simulink library "lib_ares"  (R2020a)
settings: Solver=VariableStepAuto  StartTime=0.0  StopTime=10.0  RelTol=1e-3
undefined symbols (not defined in the file or in its folder): DiscIntNeverNeededParam
libraries: simulink x9, $bdroot x6
(part 1 of 2)
settings Model: Creator=geiger_br  LastModifiedBy=geiger_br

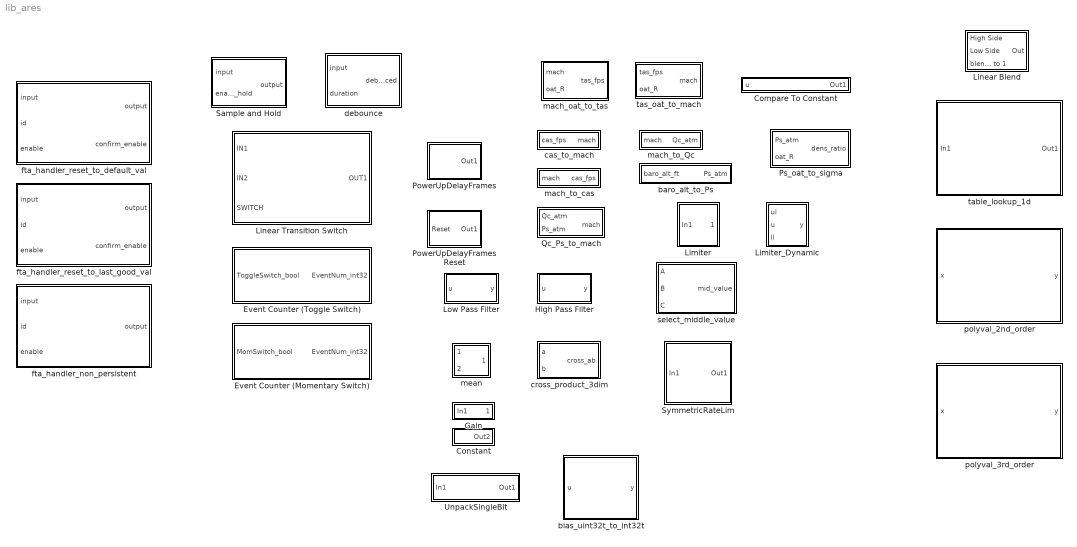
== system lib_ares ==
  Compare To Constant : Subsystem  mask{constval=0}
      mask prompts: constval "Constant:"
      mask init:
      | % Get the mask object
      | mo = get_param(gcb,'MaskObject');
      | % Get the text object
      | % tc = mo.getDialogControl('TextControl');
      | % Change the string
      | % tc.Prompt = mo.Parameters(1).Value;
      | 
      | prm_str = mo.Parameters(1).Value;
      mask Display:
      | if isnan(str2double(prm_str))
      |     fprintf('== %s (%d)',prm_str,int32(constval));
      | else
      |     fprintf('== %g',constval);
      | end
  Constant : Subsystem  mask(Custom Gain Block){const_param=1, const_datatype_str=Inherit: Inherit from 'Constant value', use_attr_fmt_str=on}
      mask prompts: const_param "Gain"; const_datatype_str "Data Type"; use_attr_fmt_str "Use Attributes Format String"
      mask help: Multiply the incoming signal by the gain value.
      mask init:
      | %
      | % NOTES
      | %    For this to work properly, 'Evaluate' must be off for const_param
      | %    The block evaluates here in initialization.
      | %
      | % int64 and uint64 types have been turned off in the Data Type option to
      | % ensure backwards compatibility with R2017a
      | %
      | 
      | evconst = evalin('base',const_param);
      | 
      | % get the mask object data
      | mo = get_param(gcb,'MaskObject');
      | 
      | % Check to see if this is a Parameter.
      | if strcmp(class(evconst),'Simulink.Parameter')
      |     is_parameter = true;
      |     const_value = evconst.Value;
      |     dtype = evconst.DataType;
      |     mo.Parameters(2).Enabled = 'off';
      |     mo.Parameters(2).Value = dtype;
      | else
      |     is_parameter = false;
      |     const_value = evconst;
      | %     dtype='Inherit: Inherit via internal rule';
      |     dtype = mo.Parameters(2).Value;
      |     mo.Parameters(2).Enabled = 'on';
      | end
      | 
      | % Set the gain block to the desired output datatype
      | set_param([gcb '/constant_value'],'OutDataTypeStr',dtype)
      | 
      | % Get the text of the input. If it is not just a number,
      | % set the AttributeFormatString to the text
      | p_str = mo.Parameters(1).Value;
      | if ~isnan(str2double(p_str)) 
      |     attstr = ''; % do not display if p_str is a number, we are showing the value below
      | else
      |     attstr = sprintf('%s',p_str);
      | end
      | 
      | sz=size(const_value);
      | assert(ndims(const_value)<=2,'Constants used with this block must be 1 or 2 dimensional only.')
      | if all(sz==1)
      |     const_str = sprintf('%g',const_value);
      | elseif sz(1)>1
      |     sep='; ';
      |     const_str = sprintf(['%0.4g' sep],const_value);
      |     const_str = sprintf('[%s]',const_str(1:end-length(sep)));
      | elseif sz(2)>1
      |     sep=', ';
      |     const_str = sprintf(['%0.4g' sep],const_value);
      |     const_str = sprintf('[%s]',const_str(1:end-length(sep)));
      | end
      | 
      | if use_attr_fmt_str
      |     set_param(gcb,'AttributesFormatString',attstr);
      |     kstr = sprintf('%s',const_str);
      | else
      |     set_param(gcb,'AttributesFormatString','');
      |     if ~isempty(attstr)
      |         attstr = sprintf('%s = ',attstr);
      |     end
      |     kstr = sprintf('%s%s',attstr,const_str);
      | end
      mask Display:
      | % Notes: See Initialization section.
      | 
      | text(0.5,0.45,kstr,'horizontalalignment','center','verticalalignment','base')
  Event Counter (Momentary Switch) : Subsystem
  Event Counter (Toggle Switch) : Subsystem
  Gain : Subsystem  mask(Custom Gain Block){gain_param=1, gain_datatype_str=Inherit: Inherit via internal rule, use_attr_fmt_str=on}
      mask prompts: gain_param "Gain"; gain_datatype_str "Data Type"; use_attr_fmt_str "Use Attributes Format String"
      mask help: Multiply the incoming signal by the gain value. If the gain value is a Simulink.Parameter object, the datatype will match the type defined in the parameter object.
      mask init:
      | %
      | % NOTES
      | %    For this to work properly, 'Evaluate' must be off for gain_param
      | %    The block evaluates here in initialization.
      | %
      | % int64 and uint64 types have been turned off in the Data Type option to
      | % ensure backwards compatibility with R2017a
      | %
      | 
      | evgain = evalin('base',gain_param);
      | 
      | % get the mask object data
      | mo = get_param(gcb,'MaskObject');
      | 
      | % Check to see if this is a Parameter.
      | if strcmp(class(evgain),'Simulink.Parameter')
      |     is_parameter = true;
      |     gain_value = evgain.Value;
      |     dtype = evgain.DataType;
      |     mo.Parameters(2).Enabled = 'off';
      |     mo.Parameters(2).Value = dtype;
      | else
      |     is_parameter = false;
      |     gain_value = evgain;
      | %     dtype='Inherit: Inherit via internal rule';
      |     dtype = mo.Parameters(2).Value;
      |     mo.Parameters(2).Enabled = 'on';
      | end
      | 
      | % Set the gain block to the desired output datatype
      | set_param([gcb '/const_gain_value'],'OutDataTypeStr',dtype)
      | 
      | % Get the text of the input. If it is not just a number,
      | % set the AttributeFormatString to the text
      | p_str = mo.Parameters(1).Value;
      | if ~isnan(str2double(p_str)) 
      |     attstr = ''; % do not display if p_str is a number, we are showing the value below
      | else
      |     attstr = sprintf('%s',p_str);
      | end
      | 
      | if use_attr_fmt_str
      |     set_param(gcb,'AttributesFormatString',attstr);
      |     kstr = sprintf('k = %g',gain_value);
      | else
      |     set_param(gcb,'AttributesFormatString','');
      |     if isempty(attstr)
      |         attstr = 'k';
      |     end
      |     kstr = sprintf('%s = %g',attstr,gain_value);
      | end
      | % kstr = sprintf('%s [%g]',attstr,gain_value);
      | % kstr = sprintf('%g (%s)',gain_value,attstr);
      mask Display:
      | % Notes: See Initialization section.
      | 
      | text(0.5,0.54,kstr,'horizontalalignment','center','verticalalignment','middle')
  High Pass Filter : Subsystem  mask(First order high pass filter){tau=1, k=1.0}
      mask prompts: tau "Time Constant (sec)"; k "Gain"
      mask help: A first order high pass filter with rectangular integration.
      mask Help: Enter the time constant and gain in the parameter fields.
      mask Display: dpoly(k*[1/tau 0],[1 1/tau])
  Limiter : Subsystem  mask(Limiter){max_val=1, min_val=-1}
      mask prompts: max_val "Maximum Limit:"; min_val "Minimum Limit:"
      mask help: Output y based on input u limited to be between the specified minimum and maximum values.
      mask Display:
      | %disp(sprintf('u_{max} \\rightarrow %g\nu_{min} \\rightarrow %g',max_val,min_val), 'texmode','on')
      | 
      | % disp(sprintf('y \\leq %g\ny \\geq %g',max_val,min_val), 'texmode','on')
      | 
      | %disp(sprintf('%g \\leq u \\leq %g',min_val,max_val), 'texmode','on')
      | 
      | min_prot = min(max_val,min_val);
      | max_prot = max(max_val,min_val);
      | 
      | port_label('input', 1, 'u');
      | port_label('output', 1, 'y');
      | 
      | hi=.7;
      | lo=.3;
      | d=hi-lo;
      | if (max_prot-min_prot)~=0
      |     plot(0*.18+[ .35 .65],lo+[ d d]*abs(min(0,min_prot))/(max_prot-min_prot));
      | end
      | 
      | color('blue')
      | bb=[1 1]; % this will cause all further plotting to be bold
      | plot(0*.18+[bb*0.25 0.45 .55 .75],[ bb*lo lo hi hi]);
      | 
      | text(.75,hi+0.01,sprintf('%g',max_prot),'horizontalAlignment','right','verticalAlignment','bottom');
      | text(.25,lo,sprintf('%g',min_prot),'horizontalAlignment','left','verticalAlignment','top');
  Limiter_Dynamic : Subsystem  mask(Saturation Limit (Dynamic)){}
      mask help: Limit input u to be between UL and LL inputs.
      mask Display:
      | %disp(sprintf('u_{max} \\rightarrow %g\nu_{min} \\rightarrow %g',max_val,min_val), 'texmode','on')
      | 
      | % disp(sprintf('y \\leq %g\ny \\geq %g',max_val,min_val), 'texmode','on')
      | 
      | %disp(sprintf('%g \\leq u \\leq %g',min_val,max_val), 'texmode','on')
      | 
      | port_label('input', 1, 'UL');
      | port_label('input', 2, 'u');
      | port_label('input', 3, 'LL');
      | port_label('output', 1, 'y');
      | 
      | plot(.1+[.35 .65],.1+[.8 .8]*0.5);
      | % plot(.1+[.5 .5],[.1 .9])
      | 
      | color('blue')
      | bb=[1 1]; % this will cause all further plotting to be bold
      | plot(.1+[bb*0.25 0.45 .55 .75],[bb*.2 .2 .8 .8]);
      | 
      | %text(.55,1,'UL','horizontalAlignment','right','verticalAlignment','top')
      | %text(.55,.12,'LL','horizontalAlignment','right','verticalAlignment','bottom')
  Linear Blend : Subsystem  mask(Linearly Blend Inputs){}
      mask help:
      | Given two inputs (In0 and In1) and a transition variable (s) that can vary from 0 to 1, linearly blend from In0 to In1 using the value of the transition variable.
      |
      | The transition variable is internally limited to exist betwen 0 and 1.
      |
      | When the transition variable is 0 or less, output In0; when the transition variable is greater than or equal to 1, output In1; when the transition variable is between 0 and 1 output (In1*s+In0*(1-s)).
      mask Display:
      | plot([0.05,0.65,0.65],[.165 .165 .31]) % arrow base
      | % plot([.47 .5 .53],[.3 .4 .3]) % arrow head
      | patch(.65+[0 -0.04 0.04],[.42 .3 .3]) % arrow head
      | plot([0.8 0.8],[0.47 0.77])
      | plot([0.5 0.5],[0.47,0.55])
      | text(.5,.37,'0','horizontalalignment','center')
      | text(.8,.37,'1','horizontalalignment','center')
      | text(.05,.835,'In1','verticalalignment','middle')
      | text(.05,.5,'In0','verticalalignment','middle')
      | color('blue')
      | plot([.4 .4 .4 0.5 0.8 0.9],[.5 .5 .5 .5 .835 .835]) % transition plot
  Linear Transition Switch : Subsystem  mask(Linear Transition Switch){Tblend=2}
      mask prompts: Tblend "Blend Time (sec)"
      mask help: The linear transition switch will linearaly fade from IN1 to IN2 when the SWITCH port is > 0
      mask Help: Enter the transition time in seconds in the block diagram parameter fields.
      mask Display:
      | fprintf('T_blend = %g s', Tblend)
      | 
      | port_label('input', 1, 'IN1')
      | port_label('input', 2, 'IN2')
      | port_label('input', 3, 'SWITCH')
      | port_label('output', 1, 'OUT')
  Low Pass Filter : Subsystem  mask(First order low pass filter){tau=1, k=1.0}
      mask prompts: tau "Time Constant (sec)"; k "Gain"
      mask help: A first order low pass filter with rectangular integration.
      mask Help: Enter the time constant and gain in the parameter fields.
      mask Display: dpoly(k*[1/tau],[1 1/tau])
  PowerUpDelayFrames : Subsystem  mask{Nframes=1}
      mask prompts: Nframes "Number of Frames to Wait:"
      mask init:
      | assert(Nframes>0,'Number of frames to wait must be greater than zero.');
      | assert(isa(Nframes,'numeric'));
      | 
      | 
      | mo = get_param(gcb,'MaskObject');
      | p_str = mo.Parameters(1).Value;
      | 
      | if ~isnan(str2double(p_str)) 
      |     p_str = ''; % do not display if p_str is a number, we are showing the value below
      | else
      |     p_str = sprintf(' (%s)',p_str);
      | end
      | 
      | if Nframes == 1
      |     attstr = sprintf('Wait 1 Frame%s',p_str);
      | else
      |     attstr = sprintf('Wait %d Frames%s',Nframes,p_str);
      | end
      | 
      | 
      | 
      | 
      | 
      | set_param(gcb,'AttributesFormatString',attstr);
      settings: AttributesFormatString=Wait 1 Frame
      mask Display:
      | text(0.15,0.32,'Delay','horizontalalignment','left','verticalalignment','top');
      | % text(0.2,0.3,'OFF','horizontalalignment','left','verticalalignment','bottom');
      | text(0.9,0.9,'ON','horizontalalignment','right','verticalalignment','top');
      | 
      | plot([0.15 0.6 0.6 0.9],[.32 .32 .9 .9]);
  PowerUpDelayFramesReset : Subsystem  mask(Delay N Frames with Reset){Nframes=1}
      mask prompts: Nframes "Number of Frames to Wait:"
      mask help: If Reset is false (0), output false (0) for N frames, then output true (1). If Reset is true (~0), output false (0).
      mask init: same as lib_ares/PowerUpDelayFrames
      settings: AttributesFormatString=Wait 1 Frame
      mask Display:
      | text(0.15,0.32,'Delay','horizontalalignment','left','verticalalignment','top');
      | % text(0.2,0.3,'OFF','horizontalalignment','left','verticalalignment','bottom');
      | text(0.9,0.9,'ON','horizontalalignment','right','verticalalignment','top');
      | 
      | plot([0.15 0.6 0.6 0.9],[.32 .32 .9 .9]);
      | 
      | port_label('input',1,'Reset');
  Ps_oat_to_sigma : Subsystem
  Qc_Ps_to_mach : Subsystem
  Sample and Hold : Subsystem
  SymmetricRateLim : Subsystem  mask(Limiter){ratelim_param=1}
      mask prompts: ratelim_param "Rate Limit:"
      mask help: Output y based on input u limited to be between the specified minimum and maximum values.
      mask init:
      | evratelim = evalin('base',ratelim_param);
      | 
      | % get the mask object data
      | mo = get_param(gcb,'MaskObject');
      | 
      | 
      | % Check to see if this is a Parameter.
      | if strcmp(class(evratelim),'Simulink.Parameter')
      |     is_parameter = true;
      |     ratelim = evratelim.Value;
      |     dtype = evratelim.DataType;
      | %     mo.Parameters(2).Enabled = 'off';
      | %     mo.Parameters(2).Value = dtype;
      | else
      |     is_parameter = false;
      |     ratelim = evratelim;
      | %     dtype='Inherit: Inherit via internal rule';
      | %     dtype = mo.Parameters(2).Value;
      | %     mo.Parameters(2).Enabled = 'on';
      | end
      | 
      | 
      | assert(ratelim>0,'Rate limit must be greater than zero')
      | 
      | 
      | p_str = mo.Parameters(1).Value;
      | if ~isnan(str2double(p_str)) 
      |     attstr = ''; % do not display if p_str is a number, we are showing the value below
      | else
      |     attstr = sprintf('%s',p_str);
      | end
      | 
      | set_param(gcb,'AttributesFormatString',attstr);
      mask Display:
      | port_label('input', 1, 'u');
      | port_label('output', 1, 'y');
      | 
      | color('blue')
      | bb=[1 1]; % this will cause all further plotting to be bold
      | 
      | 
      | text(.5,.05,sprintf('±%g/sec',ratelim),'horizontalalignment','center','verticalalignment','bottom')
      | 
      | yb=-.1;
      | 
      | % limited rates
      | patch([0.5 .8 .2],[.5 .2 .2]-yb,[1,.7,.7])
      | patch([0.5 .2 .8],[.5 .8 .8]-yb,[1,.7,.7])
      | 
      | % allowed rates
      | patch([0.2 .2 .5],[.2 .8 .5]-yb,[.9,1,.9])
      | patch([0.5 .8 .8],[.5 .2 .8]-yb,[.9,1,.9])
      | 
      | color('black')
      | plot([.5,.5,NaN,.15,.85],[.15 .85 NaN .5 .5]-yb); % plot grid
      | 
      | color('magenta')
      | plot([.3 .4 .4],[.3 .3 .4]-yb)
      | 
      | % plot dashed lines
      | % N=20; % must be even
      | % xd = reshape([reshape(linspace(-.3,.3,N),2,[]);NaN*zeros(1,N/2)],[],1);
      | % plot(xd+0.5,(xd*1.2)+0.5)
      | % plot(xd+0.5,(xd*1.5)+0.5)
      | 
      | 
      | % color('black')
      | % plot([.2 .8],[.2,.8])
      | 
      | 
      | xd=[-.3 .3];
      | color('red')
      | plot(xd+0.5,(xd*1)+0.5-yb)
      | plot(xd+0.5,-(xd*1)+0.5-yb)
      | 
      | color('blue')
      | % plot(xd+0.5,(xd*0.6)+0.5-yb)
      | plot(xd+0.5,(xd*0.3)+0.5-yb)
      | 
      | plot(xd+0.5,-(xd*0.6)+0.5-yb)
      | % plot(xd+0.5,-(xd*0.3)+0.5-yb)
  UnpackSingleBit : Subsystem  mask{bit_index=0}
      mask prompts: bit_index "Bit Number [zero based]"
      mask init:
      | bitmask_intval=0;
      | 
      | assert( ~ischar(bit_index), 'Bit index must be an integer.');
      | assert( bit_index>=0, 'Bit index must be >= zero.');
      | assert( mod(bit_index,1)==0, 'Bit index must be an integer');
      | 
      | bitmask_intval = 2^bit_index;
      | 
      | 
      | % bitmask_param
      | 
      | % bitmask = strtrim(bitmask_param);
      | % if all(lower(bitmask(1:2))=='0x')
      | %     bitmask = bitmask(3:end);
      | % end
      | %     
      | % assert(~isempty(bitmask),'Bit mask cannot be empty')
      | % isHexCheck = regexp(bitmask,'^[0-9abcedfABCDEF]+$')
      | % assert(~isempty(isHexCheck) && isHexCheck==1,'Bit mask must be a valid hex string.')
      | % 
      | % bitmask_intval = hex2dec(bitmask);
      mask Display:
      | mstr = sprintf('Unpack Bit %d\nMask: 0x%x',bit_index,bitmask_intval);
      | text(0.5,0.52,mstr,'horizontalalignment','center','verticalalignment','middle');
  baro_alt_to_Ps : Subsystem
  bias_uint32t_to_int32t : Subsystem
      mask Display:
      | xb=0.05;
      | plot(xb+[.25,.8],[.5,.5])
      | plot(xb+[.3,.3],[.2,.8])
      | plot(xb+[.25 .35],[.3 .3])
      | plot(xb+[.25 .35],[.7 .7])
      | plot(xb+[.7 .7],[.45 .55])
      | 
      | text(.5,.95,'uint_32 -> int_32','horizontalalignment','center')
      | 
      | text(.7,.48,'2³²-1','horizontalalignment','left','verticalalignment','top')
      | text(.29,.7,'2³¹-1','horizontalalignment','right','verticalalignment','middle')
      | text(.29,.3,'-2³¹','horizontalalignment','right','verticalalignment','middle')
      | 
      | color('blue')
      | plot(xb+[.3 .3 .7],[.3 .3,.7])
  cas_to_mach : Subsystem
  cross_product_3dim : Subsystem
  debounce : Subsystem
  fta_handler_non_persistent : Subsystem  mask(Enable Parameter via ID (Non-Persistent)){id=-1, default_value=0}
      mask prompts: id "FTA Verb ID"; default_value "Default value:"
      mask help:
      | Send input if verb ID matches and ENABLE is TRUE.
      |
      | Output the input value when [FTA Verb] and verb match and ENABLE is TRUE. When ENABLE is FALSE, output [Default Value].
      mask Display:
      | port_label('input',1,'in');
      | % port_label('input',2,'id')
      | port_label('input',2,sprintf('== FTA Verb %d',id));
      | port_label('input',3,'enable');
      | port_label('output',1,'out');
      | 
      | % text(.5,0,str,'verticalalignment','bottom','horizontalalignment','center')
      | text(.5,0,sprintf('Reset to:\nDefault Value'),'verticalalignment','bottom','horizontalalignment','center');
      | 
      | color('blue');
      | str=sprintf('FTA Verb %d\nDefault Value: %g\nNon-Persistent',id,default_value);
      | text(.5,1,str,'verticalalignment','top','horizontalalignment','center');
  fta_handler_reset_to_default_val : Subsystem  mask(Trial Parameter with Reset to Default Value){id=-1, trial_time=1, default_value=0}
      mask prompts: id "FTA Verb ID"; trial_time "Trial time (sec):"; default_value "Default value:"
      mask help:
      | Send input with auto-reset to default if disable before timeout
      |
      | Output the input value when [FTA Verb] and verb match and ENABLE is TRUE. When this occurs, a timer starts counting for [Trial Time] seconds. If ENABLE becomes false before the [Trial Time] has expired, reset output to the [Default Value]. If ENABLE becomes false after [Trial Time] has elapsed, the value of the input at this time will continue to be sent to the output.
      |
      | This subsystem can always be reset to the default value by sending an ENABLE pulse that is shorter than the trial time (pulse is FALSE then TRUE then FALSE).
      mask Display:
      | port_label('input',1,'in');
      | % port_label('input',2,'id')
      | port_label('input',2,sprintf('== FTA Verb %d',id));
      | port_label('input',3,'enable');
      | port_label('output',1,'out');
      | port_label('output',2,'confirm');
      | 
      | % text(.5,0,str,'verticalalignment','bottom','horizontalalignment','center')
      | text(.5,0,sprintf('Reset to:\nDefault Value'),'verticalalignment','bottom','horizontalalignment','center');
      | 
      | color('blue');
      | str=sprintf('FTA Verb %d\nDefault Value: %g\nTrial Time: %g sec',id,default_value,trial_time);
      | text(.5,1,str,'verticalalignment','top','horizontalalignment','center');
  fta_handler_reset_to_last_good_val : Subsystem  mask(Trial Parameter with Reset to Last Good Value){id=-1, trial_time=1, default_value=0}
      mask prompts: id "FTA Verb ID"; trial_time "Trial time (sec):"; default_value "Default value:"
      mask help:
      | Send input with auto-reset to default or last good value if disable before timeout.
      |
      | Output the input value when [FTA Verb] and verb match and ENABLE is TRUE. When this occurs, a timer starts counting for [Trial Time] seconds. If ENABLE becomes false before the [Trial Time] has expired, reset output to the [Default Value]. If ENABLE becomes false after [Trial Time] has elapsed, the value of the input at this time will continue to be sent to the output. This value also becomes the [Default Value].
      |
      | This subsystem will update the [Default Value] when an input value is held for longer than the [Trial Time]. After this update occurs, any reset action will use the new [Default Value] until another input value is held for longer than the [Trial Time].
      mask Display:
      | port_label('input',1,'in');
      | % port_label('input',2,'id')
      | port_label('input',2,sprintf('== FTA Verb %d',id));
      | port_label('input',3,'enable');
      | port_label('output',1,'out');
      | port_label('output',2,'confirm');
      | 
      | color('red');
      | text(.25,0,sprintf('Reset Behavior:\n  Initial: %g\n  Then: Last Good Value',default_value),'verticalalignment','bottom','horizontalalignment','left');
      | 
      | color('blue');
      | str=sprintf('FTA Verb %d\nDefault Value: %g\nTrial Time: %g sec',id,default_value,trial_time);
      | text(.5,1,str,'verticalalignment','top','horizontalalignment','center');
  mach_oat_to_tas : Subsystem
  mach_to_Qc : Subsystem
  mach_to_cas : Subsystem
  mean : Subsystem
      mask Display: disp('mean')
  polyval_2nd_order : Subsystem  mask(Polyval 2nd Order){p=[1,2,-0.5], x_min=-1, x_max=1}
      mask prompts: p "Poly. Coeffs:"; x_min "X Min:"; x_max "X Max:"
      mask help:
      | Calculates the 2nd order polynomial from coefficients p and inputs x. p must be length 3. See also 'polyval' function. x is limited to the specified min and max.
      |
      |          y = p1 * x^2 + p2 * x + p3
      mask init:
      | % Get the mask object
      | mo = get_param(gcb,'MaskObject');
      | p_str = mo.Parameters(1).Value;
      | 
      | % Remove the useless '.Value' if we had to use it.
      | if strcmp(p_str(end-5:end),'.Value')
      |     p_str = p_str(1:end-6);
      | end
      | 
      | set_param(gcb,'AttributesFormatString',sprintf('p=%s (clip)',p_str));
      | 
      | assert(length(p)==3,'Length of p must be 3');
      | assert(length(x_min)==1, 'Length of x_min must be 1');
      | assert(length(x_max)==1, 'Length of x_max must be 1');
      settings: AttributesFormatString=p=[1,2,-0.5] (clip)
      mask Display:
      | port_label('input',1,'x')
      | port_label('output',1,'y')
      | 
      | 
      | 
      | pos=get_param(gcb,'Position');
      | blk_xpx = pos(3)-pos(1); % horz width of block in pixels
      | blk_ypx = pos(4)-pos(2); % vert width of block in pixels
      | 
      | xlo=min(x_min,x_max); % minimum x-value in data
      | xhi=max(x_min,x_max); % maximum x-value in data
      | 
      | xdat = linspace(xlo,xhi,15); % sample x input data for plotting
      | ydat = polyval(p,xdat);
      | 
      | ylo=min(ydat); % minimum y-value in data
      | yhi=max(ydat); % maximum y-value in data
      | 
      | % these are normalized coordinates for drawing a box inside the block mask
      | % the normalized size of this box is controlled by xmarg & ymarg
      | xbrdr=[0,0,1,1,0,0]; % these are the plot border lines (to be scaled later). Note repeated first values to plot in bold.
      | ybrdr=[0,0,0,1,1,0];
      | xmid=[ 0.50,0.50, nan, -0.01,0.03, nan, 0.50,0.50, nan, 0.97,1.01];
      | ymid=[-0.01,0.03, nan,  0.50,0.50, nan, 0.97,1.01, nan, 0.50,0.50];
      | xzgrd=([xlo,xhi, nan,   0,  0]-xlo)/(xhi-xlo); % x-coords of grid line at zero
      | yzgrd=([  0,  0, nan, ylo,yhi]-ylo)/(yhi-ylo); % y-coords of grid line at zero
      | 
      | 
      | xmarg = [18 32]/blk_xpx; % left and right margin (px normalized)
      | ymarg = [18  5]/blk_ypx; % bottom and top margin (px normalized)
      | 
      | xfac = max(1 - sum(xmarg),.3); % width of mask art
      | yfac= max(1 - sum(ymarg),.3); % height of mask art
      | xb = xmarg(1);  % left side location of mask art
      | yb = ymarg(1); % bottom side location of mask art
      | 
      | color('black')
      | if xzgrd(4)>0.01 && xzgrd(4)<0.99
      |     patch(xb+xfac*xzgrd(4:5),yb+yfac*yzgrd(4:5),.8*[1,1,1]); % can fake color in lines with this
      | end
      | if yzgrd(1)>0.01 && yzgrd(1)<0.99
      |     patch(xb+xfac*xzgrd(1:2),yb+yfac*yzgrd(1:2),.8*[1,1,1]); % can fake color in lines with this
      | end
      | 
      | % patch(xb+xfac*xzgrd,yb+yfac*yzgrd,.6*[1,1,1]) % can fake color in lines with this
      | plot(xb+xfac*xbrdr,yb+yfac*ybrdr); % Draw the border box around the plot
      | plot(xb+xfac*xmid,yb+yfac*ymid); % Draw the mid-point ticks on the border box
      | 
      | 
      | text(xb+xfac*0.5,yb+yfac*0,'x','verticalalignment','top','horizontalalignment','center');
      | text(xb+xfac*1,yb+yfac*0.5,' y','verticalalignment','base','horizontalalignment','left');
      | 
      | color('magenta');
      | x_data_line = xb+xfac*([ xdat]-xlo)/(xhi-xlo);  x_data_line  =[x_data_line(1) x_data_line]; % these repeated first points draw bold lines (sometimes?)
      | y_data_line = yb+yfac*([ ydat]-ylo)/(yhi-ylo);  y_data_line = [y_data_line(1) y_data_line];
      | plot( x_data_line,  y_data_line);
      | 
      | color('blue');
      | text(xb+xfac*0,yb+yfac*0,sprintf('%0.4g',xlo),'verticalalignment','top','horizontalalignment','left');
      | text(xb+xfac*1,yb+yfac*0,sprintf('%0.4g  ',xhi),'verticalalignment','top','horizontalalignment','center');
      | text(xb+xfac*1,yb+yfac*0,sprintf(' %0.4g',ylo),'verticalalignment','base','horizontalalignment','left');
      | text(xb+xfac*1,yb+yfac*1,sprintf(' %0.4g',yhi),'verticalalignment','middle','horizontalalignment','left');
  polyval_3rd_order : Subsystem  mask(Polyval 3rd Order){p=[2,1,1,-0.5], x_min=-1, x_max=1}
      mask prompts: p "Poly. Coeffs:"; x_min "X Min:"; x_max "X Max:"
      mask help:
      | Calculates the 3rd order polynomial from coefficients p and inputs x. p must be length 4. See also 'polyval' function. x is limited to the specified min and max.
      |
      |      y = p1 * x^3 + p2 * x^2 + p3 * x + p4
      mask init:
      | % Get the mask object
      | mo = get_param(gcb,'MaskObject');
      | p_str = mo.Parameters(1).Value;
      | 
      | % Remove the useless '.Value' if we had to use it.
      | if strcmp(p_str(end-5:end),'.Value')
      |     p_str = p_str(1:end-6);
      | end
      | 
      | set_param(gcb,'AttributesFormatString',sprintf('p=%s (clip)',p_str));
      | 
      | assert(length(p)==4,'Length of p must be 4');
      | assert(length(x_min)==1, 'Length of x_min must be 1');
      | assert(length(x_max)==1, 'Length of x_max must be 1');
      settings: AttributesFormatString=p=[2,1,1,-0.5] (clip)
      mask Display:
      | port_label('input',1,'x')
      | port_label('output',1,'y')
      | 
      | 
      | 
      | pos=get_param(gcb,'Position');
      | blk_xpx = pos(3)-pos(1); % horz width of block in pixels
      | blk_ypx = pos(4)-pos(2); % vert width of block in pixels
      | 
      | xlo=min(x_min,x_max); % minimum x-value in data
      | xhi=max(x_min,x_max); % maximum x-value in data
      | 
      | xdat = linspace(xlo,xhi,15); % sample x input data for plotting
      | ydat = polyval(p,xdat);
      | 
      | ylo=min(ydat); % minimum y-value in data
      | yhi=max(ydat); % maximum y-value in data
      | 
      | % these are normalized coordinates for drawing a box inside the block mask
      | % the normalized size of this box is controlled by xmarg & ymarg
      | xbrdr=[0,0,1,1,0,0]; % these are the plot border lines (to be scaled later). Note repeated first values to plot in bold.
      | ybrdr=[0,0,0,1,1,0];
      | xmid=[ 0.50,0.50, nan, -0.01,0.03, nan, 0.50,0.50, nan, 0.97,1.01];
      | ymid=[-0.01,0.03, nan,  0.50,0.50, nan, 0.97,1.01, nan, 0.50,0.50];
      | xzgrd=([xlo,xhi, nan,   0,  0]-xlo)/(xhi-xlo); % x-coords of grid line at zero
      | yzgrd=([  0,  0, nan, ylo,yhi]-ylo)/(yhi-ylo); % y-coords of grid line at zero
      | 
      | 
      | xmarg = [18 32]/blk_xpx; % left and right margin (px normalized)
      | ymarg = [18  5]/blk_ypx; % bottom and top margin (px normalized)
      | 
      | xfac = max(1 - sum(xmarg),.3); % width of mask art
      | yfac= max(1 - sum(ymarg),.3); % height of mask art
      | xb = xmarg(1);  % left side location of mask art
      | yb = ymarg(1); % bottom side location of mask art
      | 
      | color('black')
      | if xzgrd(4)>0.01 && xzgrd(4)<0.99
      |     patch(xb+xfac*xzgrd(4:5),yb+yfac*yzgrd(4:5),.8*[1,1,1]); % can fake color in lines with this
      | end
      | if yzgrd(1)>0.01 && yzgrd(1)<0.99
      |     patch(xb+xfac*xzgrd(1:2),yb+yfac*yzgrd(1:2),.8*[1,1,1]); % can fake color in lines with this
      | end
      | % patch(xb+xfac*xzgrd,yb+yfac*yzgrd,.6*[1,1,1]) % can fake color in lines with this
      | 
      | color('black')
      | plot(xb+xfac*xbrdr,yb+yfac*ybrdr); % Draw the border box around the plot
      | plot(xb+xfac*xmid,yb+yfac*ymid); % Draw the mid-point ticks on the border box
      | 
      | 
      | text(xb+xfac*0.5,yb+yfac*0,'x','verticalalignment','top','horizontalalignment','center');
      | text(xb+xfac*1,yb+yfac*0.5,' y','verticalalignment','base','horizontalalignment','left');
      | 
      | color('magenta');
      | x_data_line = xb+xfac*([ xdat]-xlo)/(xhi-xlo);  x_data_line  =[x_data_line(1) x_data_line]; % these repeated first points draw bold lines (sometimes?)
      | y_data_line = yb+yfac*([ ydat]-ylo)/(yhi-ylo);  y_data_line = [y_data_line(1) y_data_line];
      | plot( x_data_line,  y_data_line);
      | 
      | color('blue');
      | text(xb+xfac*0,yb+yfac*0,sprintf('%0.4g',xlo),'verticalalignment','top','horizontalalignment','left');
      | text(xb+xfac*1,yb+yfac*0,sprintf('%0.4g  ',xhi),'verticalalignment','top','horizontalalignment','center');
      | text(xb+xfac*1,yb+yfac*0,sprintf(' %0.4g',ylo),'verticalalignment','base','horizontalalignment','left');
      | text(xb+xfac*1,yb+yfac*1,sprintf(' %0.4g',yhi),'verticalalignment','middle','horizontalalignment','left');
  select_middle_value : Subsystem
  table_lookup_1d : Subsystem  mask(Table Lookup (1D)){xdat=[-15,5,10,20], ydat=[15,2,4,-10]}
      mask prompts: xdat "x data:"; ydat "y data:"
      mask help: Performs a 1-dimensional table lookup. Out of range values are clamped at the first and last value of y data.
      mask init:
      | % Get the mask object
      | mo = get_param(gcb,'MaskObject');
      | x_str = mo.Parameters(1).Value;
      | y_str = mo.Parameters(2).Value;
      | 
      | % Remove the useless '.Value' if we had to use it.
      | if strcmp(x_str(end-5:end),'.Value')
      |     x_str = x_str(1:end-6);
      | end
      | 
      | assert(~isempty(xdat) && ~isempty(ydat), 'X and Y input data must not be empty.')
      | assert(length(xdat)>1 && length(ydat)>1, 'X and Y input data must be at least 2 points.')
      | assert(all(size(xdat)==size(ydat)),'X and Y input data must be the same size.')
      | assert(any(size(xdat)==1), 'X and Y input data must only be row or column vectors.')
      | 
      | 
      | % Get the text of the input. If it is not just a number,
      | % set the AttributeFormatString to the text
      | if ~isempty(str2num(x_str)) 
      |     attstr = '(clip)'; % do not display if p_str is a number, we are showing the value below
      | else
      |     attstr = sprintf('%s (clip)',x_str);
      | end
      |     
      |     
      | set_param(gcb,'AttributesFormatString',attstr);
      settings: AttributesFormatString=(clip)
      mask Display:
      | port_label('input',1,'x')
      | port_label('output',1,'y')
      | 
      | 
      | pos=get_param(gcb,'Position');
      | blk_xpx = pos(3)-pos(1); % horz width of block in pixels
      | blk_ypx = pos(4)-pos(2); % vert width of block in pixels
      | 
      | 
      | xlo=min(xdat); % minimum x-value in data
      | xhi=max(xdat); % maximum x-value in data
      | ylo=min(ydat); % minimum y-value in data
      | yhi=max(ydat); % maximum y-value in data
      | 
      | % these are normalized coordinates for drawing a box inside the block mask
      | % the normalized size of this box is controlled by xmarg & ymarg
      | xbrdr=[0,0,1,1,0,0]; % these are the plot border lines (to be scaled later). Note repeated first values to plot in bold.
      | ybrdr=[0,0,0,1,1,0];
      | xmid=[ 0.50,0.50, nan, -0.01,0.03, nan, 0.50,0.50, nan, 0.97,1.01];
      | ymid=[-0.01,0.03, nan,  0.50,0.50, nan, 0.97,1.01, nan, 0.50,0.50];
      | xzgrd=([xlo,xhi, nan,   0,  0]-xlo)/(xhi-xlo); % x-coords of grid line at zero
      | yzgrd=([  0,  0, nan, ylo,yhi]-ylo)/(yhi-ylo); % y-coords of grid line at zero
      | 
      | xmarg = [17 25]/blk_xpx; % left and right margin (px normalized)
      | ymarg = [15  5]/blk_ypx; % bottom and top margin (px normalized)
      | 
      | xfac = max(1 - sum(xmarg),.3); % width of mask art
      | yfac= max(1 - sum(ymarg),.3); % height of mask art
      | xb = xmarg(1);  % left side location of mask art
      | yb = ymarg(1); % bottom side location of mask art
      | 
      | 
      | color('black')
      | if xzgrd(4)>0.01 && xzgrd(4)<0.99
      |     patch(xb+xfac*xzgrd(4:5),yb+yfac*yzgrd(4:5),.8*[1,1,1]); % can fake color in lines with this
      | end
      | if yzgrd(1)>0.01 && yzgrd(1)<0.99
      |     patch(xb+xfac*xzgrd(1:2),yb+yfac*yzgrd(1:2),.8*[1,1,1]); % can fake color in lines with this
      | end
      | % patch(xb+xfac*xzgrd,yb+yfac*yzgrd,.6*[1,0,1]) % can fake color in lines with this
      | 
      | color('black')
      | plot(xb+xfac*xbrdr,yb+yfac*ybrdr);% Draw the border box around the plot
      | plot(xb+xfac*xmid,yb+yfac*ymid); % Draw the mid-point ticks on the border box
      | 
      | text(xb+xfac*0.5,yb+yfac*0,'x','verticalalignment','top','horizontalalignment','center');
      | text(xb+xfac*1,yb+yfac*0.5,' y','verticalalignment','base','horizontalalignment','left');
      | 
      | color('magenta');
      | x_data_line = xb+xfac*([ xdat]-xlo)/(xhi-xlo);  x_data_line  =[x_data_line(1) x_data_line]; % these repeated first points draw bold lines (sometimes?)
      | y_data_line = yb+yfac*([ ydat]-ylo)/(yhi-ylo);  y_data_line = [y_data_line(1) y_data_line];
      | plot( x_data_line,  y_data_line);
      | 
      | color('blue');
      | text(xb+xfac*0,yb+yfac*0,sprintf('%0.4g',xlo),'verticalalignment','top','horizontalalignment','left');
      | text(xb+xfac*1,yb+yfac*0,sprintf('%0.4g  ',xhi),'verticalalignment','top','horizontalalignment','center');
      | text(xb+xfac*1,yb+yfac*0,sprintf(' %0.4g',ylo),'verticalalignment','base','horizontalalignment','left');
      | text(xb+xfac*1,yb+yfac*1,sprintf(' %0.4g',yhi),'verticalalignment','middle','horizontalalignment','left');
  tas_oat_to_mach : Subsystem

== system lib_ares/Compare To Constant ==
  u : Inport
  Constant5 : Constant  Value=constval
  Data Type Conversion Inherited : simulink/Signal Attributes/Data Type Conversion Inherited  ConvertRealWorld=Real World Value  DoSatur=off
      settings: SourceProductBaseCode=SL
  Relational Operator4 : RelationalOperator  Operator===  OutDataTypeStr=boolean  RndMeth=Simplest
  Out1 : Outport
  wires:
  Data Type Conversion Inherited/1 -> Relational Operator4/2
  u/1 -> Data Type Conversion Inherited/2
  Constant5/1 -> Data Type Conversion Inherited/1, Relational Operator4/1
  Relational Operator4/1 -> Out1/1

== system lib_ares/Constant ==
  constant_value : Constant  Value=const_value
  Out2 : Outport
  wires:
  constant_value/1 -> Out2/1

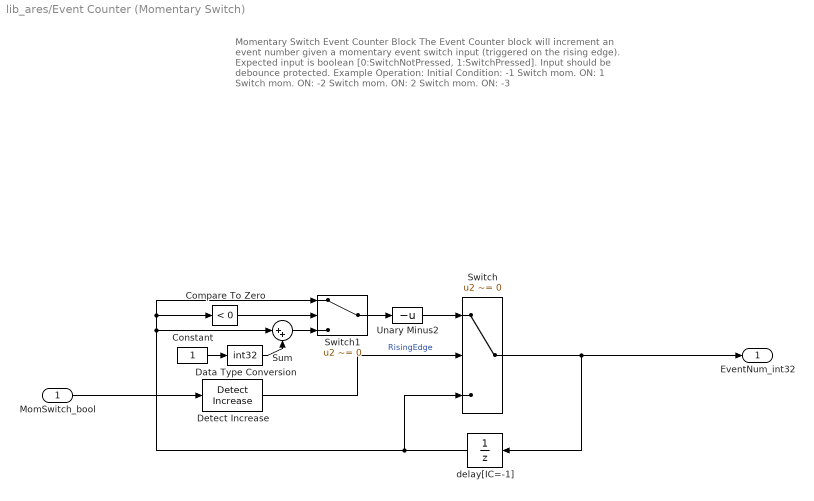
== system lib_ares/Event Counter (Momentary Switch) ==
  note: Momentary Switch Event Counter Block
      |
      | The Event Counter block will increment an event number given a momentary event switch input (triggered on the rising edge). Expected input is boolean [0:SwitchNotPressed, 1:SwitchPressed].
      |
      | Input should be debounce protected.
      |
      | Example Operation:
      | Initial Condition: -1
      | Switch mom. ON: 1
      | Switch mom. ON: -2
      | Switch mom. ON: 2
      | Switch mom. ON: -3
  MomSwitch_bool : Inport  OutDataTypeStr=boolean
  Compare To Zero : simulink/Logic and Bit Operations/Compare To Zero  relop=<  OutDataTypeStr=boolean
  Constant : Constant  OutDataTypeStr=Inherit: Inherit via back propagation
  Data Type Conversion : DataTypeConversion  OutDataTypeStr=int32
  Detect Increase : simulink/Logic and Bit Operations/Detect Increase  vinit=0.0  OutDataTypeStr=boolean
  Sum : Sum  Inputs=|++
  Switch : Switch  Criteria=u2 ~= 0
  Switch1 : Switch  Criteria=u2 ~= 0
  Unary Minus2 : UnaryMinus
  delay[IC=-1] : UnitDelay  InitialCondition=-1  SampleTime=-1  HasFrameUpgradeWarning=on
  EventNum_int32 : Outport  OutDataTypeStr=int32  VectorParamsAs1DForOutWhenUnconnected=off
  wires:
  MomSwitch_bool/1 -> Detect Increase/1
  Detect Increase/1 -> Switch/2  "RisingEdge"
  Compare To Zero/1 -> Switch1/2
  Constant/1 -> Data Type Conversion/1
  Switch/1 -> EventNum_int32/1, delay[IC=-1]/1
  Unary Minus2/1 -> Switch/1
  Sum/1 -> Switch1/3
  Switch1/1 -> Unary Minus2/1
  Data Type Conversion/1 -> Sum/2
  delay[IC=-1]/1 -> Switch/3, Switch1/1, Compare To Zero/1, Sum/1

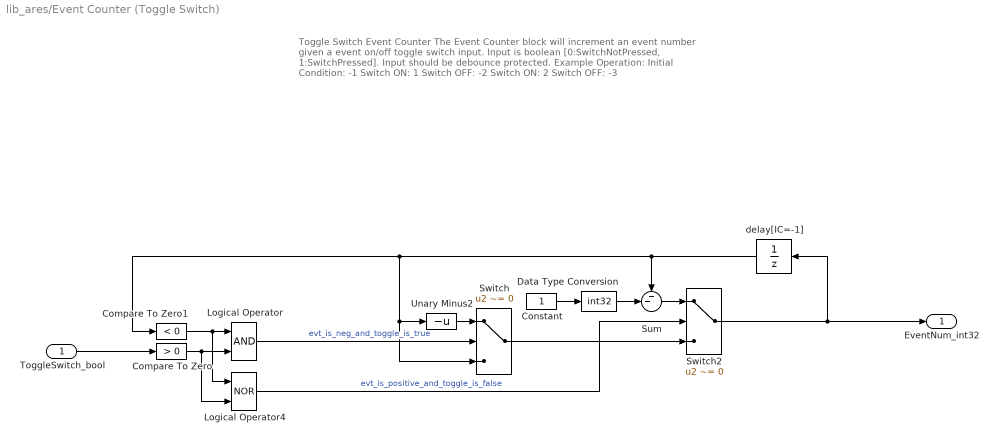
== system lib_ares/Event Counter (Toggle Switch) ==
  note: Toggle Switch Event Counter
      |
      | The Event Counter block will increment an event number given a event on/off toggle switch input. Input is boolean [0:SwitchNotPressed, 1:SwitchPressed].
      |
      | Input should be debounce protected.
      |
      | Example Operation:
      | Initial Condition: -1
      | Switch ON: 1
      | Switch OFF: -2
      | Switch ON: 2
      | Switch OFF: -3
  ToggleSwitch_bool : Inport  OutDataTypeStr=boolean
  Compare To Zero : simulink/Logic and Bit Operations/Compare To Zero  relop=>  OutDataTypeStr=boolean
  Compare To Zero1 : simulink/Logic and Bit Operations/Compare To Zero  relop=<  OutDataTypeStr=boolean
  Constant : Constant  OutDataTypeStr=Inherit: Inherit via back propagation
  Data Type Conversion : DataTypeConversion  OutDataTypeStr=int32
  Logical Operator : Logic  AllPortsSameDT=off  OutDataTypeStr=boolean
  Logical Operator4 : Logic  Operator=NOR  AllPortsSameDT=off  OutDataTypeStr=boolean
  Sum : Sum  Inputs=--|
  Switch : Switch  Criteria=u2 ~= 0
  Switch2 : Switch  Criteria=u2 ~= 0
  Unary Minus2 : UnaryMinus
  delay[IC=-1] : UnitDelay  InitialCondition=-1  SampleTime=-1  HasFrameUpgradeWarning=on
  EventNum_int32 : Outport  OutDataTypeStr=int32  VectorParamsAs1DForOutWhenUnconnected=off
  wires:
  Switch2/1 -> delay[IC=-1]/1, EventNum_int32/1
  Sum/1 -> Switch2/1
  Data Type Conversion/1 -> Sum/2
  ToggleSwitch_bool/1 -> Compare To Zero/1
  Switch/1 -> Switch2/3
  Unary Minus2/1 -> Switch/1
  Logical Operator/1 -> Switch/2  "evt_is_neg_and_toggle_is_true"
  Compare To Zero/1 -> Logical Operator4/2, Logical Operator/2
  Constant/1 -> Data Type Conversion/1
  Compare To Zero1/1 -> Logical Operator4/1, Logical Operator/1
  Logical Operator4/1 -> Switch2/2  "evt_is_positive_and_toggle_is_false"
  delay[IC=-1]/1 -> Compare To Zero1/1, Switch/3, Unary Minus2/1, Sum/1

== system lib_ares/Gain ==
  In1 : Inport
  const_gain_value : Gain  Gain=gain_value
  Out2 : Outport
  wires:
  In1/1 -> const_gain_value/1
  const_gain_value/1 -> Out2/1

== system lib_ares/High Pass Filter ==
  u : Inport
  Discrete-Time Integrator : DiscreteIntegrator  SampleTime=-1  ICPrevOutput=DiscIntNeverNeededParam  ICPrevScaledInput=DiscIntNeverNeededParam
  Gain1 : Gain  Gain=1/tau
  Gain2 : Gain  Gain=k
  Sum3 : Sum  Inputs=|+-
  y : Outport
  wires:
  Sum3/1 -> Gain1/1
  Discrete-Time Integrator/1 -> Sum3/2  "y_filt"
  Gain1/1 -> y/1, Discrete-Time Integrator/1
  Gain2/1 -> Sum3/1
  u/1 -> Gain2/1

== system lib_ares/Limiter ==
  In1 : Inport
  Constant : Constant  Value=max_val  OutDataTypeStr=Inherit: Inherit via back propagation
  Constant2 : Constant  Value=min_val  OutDataTypeStr=Inherit: Inherit via back propagation
  Data Type Duplicate : DataTypeDuplicate  DisableCoverage=on
  MinMax1 : MinMax  Inputs=2
  MinMax2 : MinMax  Function=max  Inputs=2
  MinMax3 : MinMax  Inputs=2
  MinMax4 : MinMax  Function=max  Inputs=2
  Out1 : Outport
  wires:
  MinMax1/1 -> MinMax2/1
  Constant/1 -> MinMax4/1, MinMax3/1
  In1/1 -> Data Type Duplicate/1, MinMax1/1
  MinMax2/1 -> Data Type Duplicate/2, Out1/1
  Constant2/1 -> MinMax4/2, MinMax3/2
  MinMax4/1 -> MinMax1/2
  MinMax3/1 -> MinMax2/2

== system lib_ares/Limiter_Dynamic ==
  ul : Inport
  u : Inport  Port=2
  ll : Inport  Port=3
  Data Type Duplicate : DataTypeDuplicate  DisableCoverage=on
  MinMax1 : MinMax  Inputs=2
  MinMax2 : MinMax  Function=max  Inputs=2
  MinMax3 : MinMax  Inputs=2
  MinMax4 : MinMax  Function=max  Inputs=2
  y : Outport
  wires:
  MinMax2/1 -> Data Type Duplicate/2, y/1
  u/1 -> Data Type Duplicate/1, MinMax1/1
  MinMax1/1 -> MinMax2/1
  ul/1 -> MinMax4/1, MinMax3/1
  ll/1 -> MinMax4/2, MinMax3/2
  MinMax4/1 -> MinMax1/2
  MinMax3/1 -> MinMax2/2

== system lib_ares/Linear Blend ==
  High Side : Inport
  Low Side : Inport  Port=2
  blend 0 to 1 : Inport  Port=3
  Constant5 : Constant  OutDataTypeStr=Inherit: Inherit via back propagation
  Limit 0 to 1 : Saturate  UpperLimit=1  LowerLimit=0
  Sum : Sum  Inputs=|++
  Sum22 : Sum  Inputs=+-|
  high side : Product
  low side : Product
  Out : Outport
  wires:
  low side/1 -> Sum/2
  high side/1 -> Sum/1
  Constant5/1 -> Sum22/1
  Sum22/1 -> low side/1
  blend 0 to 1/1 -> Limit 0 to 1/1
  Sum/1 -> Out/1
  High Side/1 -> high side/1
  Low Side/1 -> low side/2
  Limit 0 to 1/1 -> Sum22/2, high side/2

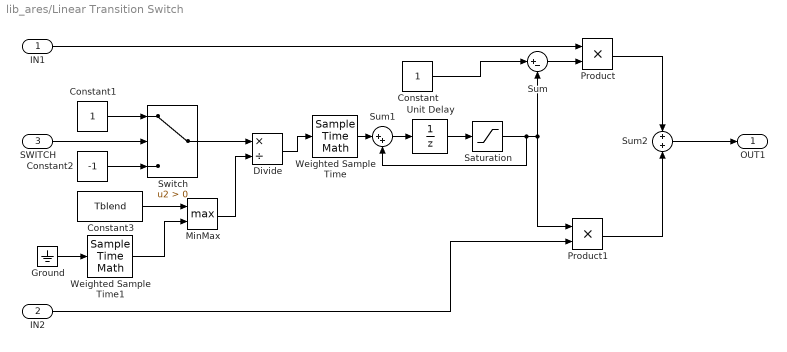
== system lib_ares/Linear Transition Switch ==
  IN1 : Inport
  IN2 : Inport  Port=2
  SWITCH : Inport  Port=3
  Constant : Constant  OutDataTypeStr=Inherit: Inherit via back propagation
  Constant1 : Constant  OutDataTypeStr=Inherit: Inherit via back propagation
  Constant2 : Constant  Value=-1  OutDataTypeStr=Inherit: Inherit via back propagation
  Constant3 : Constant  Value=Tblend  OutDataTypeStr=Inherit: Inherit via back propagation
  Divide : Product  Inputs=*/
  Ground : Ground
  MinMax : MinMax  Function=max  Inputs=2
  Product : Product
  Product1 : Product
  Saturation : Saturate  UpperLimit=1  LowerLimit=0
  Sum : Sum  Inputs=|+-
  Sum1 : Sum  Inputs=|++
  Sum2 : Sum  Inputs=+|+
  Switch : Switch  Criteria=u2 > Threshold
  Unit Delay : UnitDelay  SampleTime=-1  HasFrameUpgradeWarning=on
  Weighted Sample Time : SampleTimeMath  TsampMathOp=*
  Weighted Sample Time1 : SampleTimeMath  TsampMathOp=Ts Only
  OUT1 : Outport  VectorParamsAs1DForOutWhenUnconnected=off
  wires:
  Unit Delay/1 -> Saturation/1
  Sum1/1 -> Unit Delay/1
  Weighted Sample Time/1 -> Sum1/1
  SWITCH/1 -> Switch/2
  IN1/1 -> Product/1
  IN2/1 -> Product1/2
  Sum2/1 -> OUT1/1
  Product1/1 -> Sum2/2
  Constant1/1 -> Switch/1
  Constant2/1 -> Switch/3
  Switch/1 -> Divide/1
  Divide/1 -> Weighted Sample Time/1
  Constant3/1 -> MinMax/1
  Saturation/1 -> Product1/1, Sum/2, Sum1/2
  Constant/1 -> Sum/1
  Sum/1 -> Product/2
  Product/1 -> Sum2/1
  Weighted Sample Time1/1 -> MinMax/2
  Ground/1 -> Weighted Sample Time1/1
  MinMax/1 -> Divide/2

== system lib_ares/Low Pass Filter ==
  u : Inport
  Discrete-Time Integrator : DiscreteIntegrator  SampleTime=-1  ICPrevOutput=DiscIntNeverNeededParam  ICPrevScaledInput=DiscIntNeverNeededParam
  Gain1 : Gain  Gain=1/tau
  Gain2 : Gain  Gain=k
  Sum3 : Sum  Inputs=|+-
  y : Outport
  wires:
  Gain1/1 -> Discrete-Time Integrator/1
  Discrete-Time Integrator/1 -> y/1, Sum3/2
  Sum3/1 -> Gain1/1
  u/1 -> Gain2/1
  Gain2/1 -> Sum3/1

== system lib_ares/PowerUpDelayFrames ==
  Delay1 (x0=0) : UnitDelay  SampleTime=-1  HasFrameUpgradeWarning=on
  Relational Operator : RelationalOperator  Operator=>  OutDataTypeStr=boolean  RndMeth=Simplest
  Sum2 : Sum  Inputs=++|
  Switch2 : Switch  Criteria=u2 ~= 0
  one : Constant  OutDataTypeStr=uint32
  wait_N_frames : Constant  Value=uint32(ceil(Nframes))  OutDataTypeStr=uint32
  Out1 : Outport
  wires:
  one/1 -> Sum2/2
  Delay1 (x0=0)/1 -> Sum2/1
  wait_N_frames/1 -> Switch2/1, Relational Operator/2
  Switch2/1 -> Delay1 (x0=0)/1
  Sum2/1 -> Switch2/3, Relational Operator/1
  Relational Operator/1 -> Switch2/2, Out1/1

== system lib_ares/PowerUpDelayFramesReset ==
  Reset : Inport  OutDataTypeStr=boolean
  Delay1 (x0=0) : UnitDelay  SampleTime=-1  HasFrameUpgradeWarning=on
  Relational Operator : RelationalOperator  Operator=>  OutDataTypeStr=boolean  RndMeth=Simplest
  Sum2 : Sum  Inputs=++|
  Switch2 : Switch  Criteria=u2 ~= 0
  Switch3 : Switch  Criteria=u2 ~= 0
  one : Constant  OutDataTypeStr=uint32
  wait_N_frames : Constant  Value=uint32(ceil(Nframes))  OutDataTypeStr=uint32
  zero : Constant  Value=0  OutDataTypeStr=uint32
  Out1 : Outport
  wires:
  Relational Operator/1 -> Out1/1, Switch2/2
  Switch3/1 -> Relational Operator/1, Switch2/3
  wait_N_frames/1 -> Switch2/1, Relational Operator/2
  Delay1 (x0=0)/1 -> Sum2/1
  one/1 -> Sum2/2
  Switch2/1 -> Delay1 (x0=0)/1
  zero/1 -> Switch3/1
  Sum2/1 -> Switch3/3
  Reset/1 -> Switch3/2

== system lib_ares/Ps_oat_to_sigma ==
  note: Calculates sigma (ratio of ambient density to sea level standard density)
      | as a function of ambient pressure in atmospheres and ambient temperature
      | in Rankine.
      |
      | rho = P/(R*T)   where
      |     P: static pressure in atmospheres
      |     T: temperature in Rankine
      |     R: gas constant for air, ft-lb/(slug-degR)
      | Ref: NASA Reference Publication 1046 (1980)
  Ps_atm : Inport
  oat_R : Inport  Port=2
  Divide1 : Product  Inputs=*/
  Divide2 : Product  Inputs=*/
  GasConstAir_ftlb_slugdegR : Constant  Value=1716.5  OutDataTypeStr=single
  Product : Product
  Sea Level Std Density slug_ft3 : Constant  Value=0.0023769  OutDataTypeStr=single
  atmo_to_psf1 : Gain  Gain=2116.217
  dens_ratio : Outport
  wires:
  atmo_to_psf1/1 -> Divide2/1  "prs_static_sel_psf"
  GasConstAir_ftlb_slugdegR/1 -> Product/2
  Product/1 -> Divide2/2
  oat_R/1 -> Product/1
  Divide2/1 -> Divide1/1  "dens_ambient_slug_ft3"
  Ps_atm/1 -> atmo_to_psf1/1
  Sea Level Std Density slug_ft3/1 -> Divide1/2
  Divide1/1 -> dens_ratio/1

== system lib_ares/Qc_Ps_to_mach ==
  note: Mach as a function of Q/Ps
      | (valid for Q/Ps < 0.8929  (Mach<1))
      |
      | NASA Reference Publication 1046, Eq.3.25 Inverted
  Qc_atm : Inport
  Ps_atm : Inport  Port=2
  Divide : Product  Inputs=*/
  Qc_Ps_to_mach : Fcn  Expr="sqrt(  5.0*( (u+1.0)^(2/7) - 1.0)  )"
  mach : Outport
  wires:
  Qc_Ps_to_mach/1 -> mach/1
  Qc_atm/1 -> Divide/1
  Ps_atm/1 -> Divide/2
  Divide/1 -> Qc_Ps_to_mach/1  "Qc_Ps"

== system lib_ares/Sample and Hold ==
  note: Track and Store Block
      |
      | always pass the first input regardless
      | of enable_hold value
      |
      | if enable_hold == false then
      |        output = input
      |
      | if enable_hold == true then
      |       save current output
      |       output=unit_delay
  input : Inport
  enable_hold : Inport  Port=2
  Constant : Constant  Value=0  OutDataTypeStr=boolean
  Logical Operator : Logic  Operator=OR  AllPortsSameDT=off  OutDataTypeStr=boolean
  Logical Operator1 : Logic  Operator=NOT  AllPortsSameDT=off  OutDataTypeStr=boolean
  Switch1 : Switch  Criteria=u2 ~= 0
  Unit Delay : UnitDelay  SampleTime=-1  HasFrameUpgradeWarning=on
  initialize_store : UnitDelay  InitialCondition=1  SampleTime=-1  HasFrameUpgradeWarning=on
  output : Outport  VectorParamsAs1DForOutWhenUnconnected=off
  wires:
  Logical Operator1/1 -> Logical Operator/2
  Logical Operator/1 -> Switch1/2
  initialize_store/1 -> Logical Operator/1
  Constant/1 -> initialize_store/1
  input/1 -> Switch1/1
  enable_hold/1 -> Logical Operator1/1
  Switch1/1 -> Unit Delay/1, output/1
  Unit Delay/1 -> Switch1/3

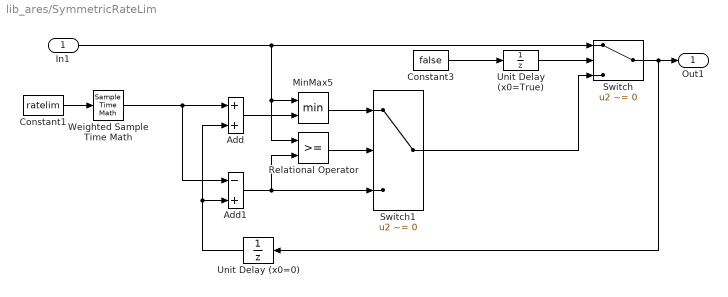
== system lib_ares/SymmetricRateLim ==
  In1 : Inport
  Add : Sum
  Add1 : Sum  Inputs=-+
  Constant1 : Constant  Value=ratelim  OutDataTypeStr=Inherit: Inherit via back propagation
  Constant3 : Constant  Value=false
  MinMax5 : MinMax  Inputs=2
  Relational Operator : RelationalOperator  OutDataTypeStr=boolean  RndMeth=Simplest
  Switch : Switch  Criteria=u2 ~= 0
  Switch1 : Switch  Criteria=u2 ~= 0
  Unit Delay (x0=0) : UnitDelay  InitialCondition=true  SampleTime=-1  HasFrameUpgradeWarning=on
  Unit Delay (x0=True) : UnitDelay  InitialCondition=true  SampleTime=-1  HasFrameUpgradeWarning=on
  Weighted Sample Time Math : SampleTimeMath  TsampMathOp=*  TsampMathImp=Offline Scaling Adjustment
  Out1 : Outport
  wires:
  Switch/1 -> Unit Delay (x0=0)/1, Out1/1
  In1/1 -> Relational Operator/1, MinMax5/1, Switch/1
  Constant1/1 -> Weighted Sample Time Math/1
  Unit Delay (x0=True)/1 -> Switch/2
  Constant3/1 -> Unit Delay (x0=True)/1
  MinMax5/1 -> Switch1/1
  Switch1/1 -> Switch/3
  Add/1 -> MinMax5/2
  Weighted Sample Time Math/1 -> Add1/1, Add/1
  Add1/1 -> Relational Operator/2, Switch1/3
  Relational Operator/1 -> Switch1/2
  Unit Delay (x0=0)/1 -> Add/2, Add1/2

== system lib_ares/UnpackSingleBit ==
  In1 : Inport
  Bitwise Operator7 : simulink/Logic and Bit Operations/Bitwise Operator  logicop=AND  UseBitMask=on  BitMask=bitmask_intval  BitMaskRealWorld=Stored Integer
  Data Type Conversion34 : DataTypeConversion  OutDataTypeStr=boolean
  Out1 : Outport  OutDataTypeStr=boolean
  wires:
  Data Type Conversion34/1 -> Out1/1
  Bitwise Operator7/1 -> Data Type Conversion34/1
  In1/1 -> Bitwise Operator7/1
